simulink model "sim6"  (R2023b)
settings: Solver=VariableStepAuto  StartTime=0.0  StopTime=20  RelTol=1e-3
settings Model: Creator=anura  LastModifiedBy=anura

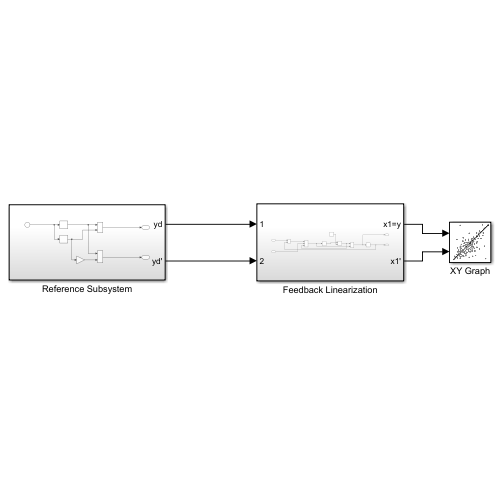
[thumbnail: Simulink's stored preview of the top-level diagram]
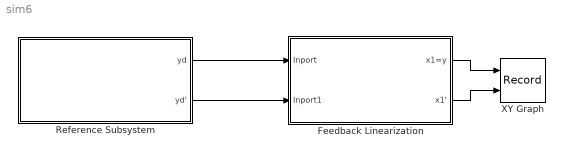
== system sim6 ==
  Feedback Linearization : Subsystem
  Reference Subsystem : Subsystem
  XY Graph : Record  FileSettingsInternal="{\"entries\":[{\"content\":{\"excelSettings\":{\"content\":{},\"type\":\"Streamout.ExcelSettings\"}},\"type\":\"Streamout.FileSettingStorage\",\"uuid\":\"\"}],\"packageUris\":[\"http:\\/\\/schema.mathworks.com\\/mf0\\/streamout_blocks\\/R2020a\"],\"version\":\"1.0\"}"  Layout=[1 1]  SignalsInternal="{\"entries\":[{\"content\":{\"signals\":[{\"content\":{\"blockPath\":[],\"dimensions\":[1],\"domain\":\"\",\"lineColor\":\"#a2142f\",\"plots\":[1],\"port\":1,\"sid\":[\"\"],\"signalID\":444,\"signalName\":\"Feedback Linearization:1\"},\"type\":\"RecordBlkView.Signal\",\"uuid\":\"\"},{\"content\":{\"blockPath\":[],\"dimensions\":[1],\"domain\":\"\",\"lineColor\":\"#139fff\",\"plots\":[1],\"port\":2,\"sid\":[\"\"],\"signalID\":448,\"signalName\":\"Feedback Linearization:2\"},\"type\":\"RecordBlkView.Signal\",\"uuid\":\"\"}]},\"type\":\"RecordBlkView.InputSignals\",\"uuid\":\"\"}],\"packageUris\":[\"http:\\/\\/schema.mathworks.com\\/mf0\\/streamout_blocks\\/R2020a\"],\"version\":\"1.0\"}"  VisualizationBindings="{\"xyplotplugin\":{\"info\":[{\"series\":[{\"bindingParametersList\":[{\"parameter\":\"X-Axis\",\"signalID\":444,\"signalName\":\"Feedback Linearization:1\"},{\"parameter\":\"Y-Axis\",\"signalID\":448,\"signalName\":\"Feedback Linearization:2\"}],\"seriesID\":46414}],\"subplotID\":1}]}}"  CompatibilityTag=XY
  wires:
  Reference Subsystem/1(yd) -> Feedback Linearization/1(Inport)
  Reference Subsystem/2(yd') -> Feedback Linearization/2(Inport1)
  Feedback Linearization/1(x1=y) -> XY Graph/1
  Feedback Linearization/2(x1') -> XY Graph/2

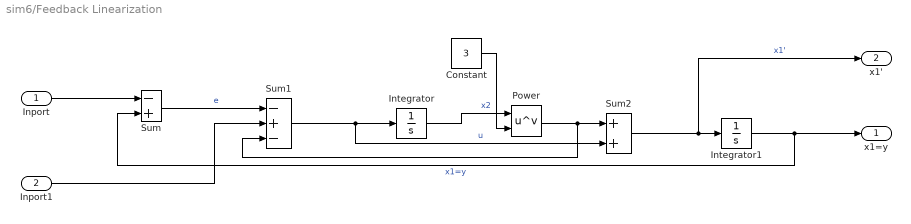
== system sim6/Feedback Linearization ==
  Inport : Inport
  Inport1 : Inport  Port=2
  Constant : Constant  Value=3
  Integrator : Integrator
  Integrator1 : Integrator
  Power : Math  Operator=pow
  Sum : Sum  Inputs=-+
  Sum1 : Sum  Inputs=-+-
  Sum2 : Sum
  x1=y : Outport
  x1' : Outport  Port=2
  wires:
  Inport/1 -> Sum/1
  Sum/1 -> Sum1/1  "e"
  Inport1/1 -> Sum1/2
  Sum1/1 -> Sum2/2, Integrator/1  "u"
  Sum2/1 -> x1'/1, Integrator1/1  "x1'"
  Integrator1/1 -> Sum/2, x1=y/1  "x1=y"
  Power/1 -> Sum1/3, Sum2/1
  Integrator/1 -> Power/1  "x2"
  Constant/1 -> Power/2

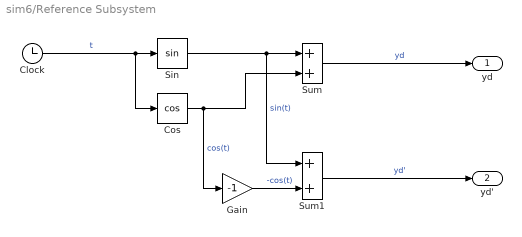
== system sim6/Reference Subsystem ==
  Clock : Clock
  Cos : Trigonometry  Operator=cos
  Gain : Gain  Gain=-1
  Sin : Trigonometry
  Sum : Sum
  Sum1 : Sum
  yd : Outport
  yd' : Outport  Port=2
  wires:
  Sin/1 -> Sum1/1, Sum/1  "sin(t)"
  Cos/1 -> Gain/1, Sum/2  "cos(t)"
  Sum/1 -> yd/1  "yd"
  Sum1/1 -> yd'/1  "yd'"
  Clock/1 -> Cos/1, Sin/1  "t"
  Gain/1 -> Sum1/2  "-cos(t)"
